simulink model "ee_asm_generator_fourier"  (R2021a)
settings: Solver=ode4  StartTime=0.0  StopTime=Wf.time(end)  FixedStep=1e-2  MaxStep=1e-4  RelTol=1e-3  EnableMultiTasking=on
PreLoadFcn:
  | SRated = 150e3; % V*A
  | VRated = 440; % V
  | FRated = 60; % Hz
  | 
  | QNominal = sin(acos(0.8))*SRated;
  | QPerPhase = QNominal / 3;
  | 
  | IPerPhase = QPerPhase/VRated;
  | Xc = VRated/IPerPhase;
  | reactiveCompensationCapacitance = 1/(2*pi*FRated*Xc);
  | 
  | clear( 'QNominal', 'QPerPhase', 'IPerPhase', 'Xc' );
StopFcn:
  | ee_addSimlogTimeStamp(bdroot)
undefined symbols (not defined in the file): g_r, H, i, J, Wf
libraries: ee_lib x8, nesl_utility x4, fl_lib x3
CloseFcn:
  | try,close(h1_ee_asm_generator),end
  | clear h1_ee_asm_generator
  | 
  | clear simlog_ee_asm_generator
  | clear logsout_ee_asm_generator
Description:
  | Three-Phase Asynchronous Wind Turbine Generator
settings Model: SimulationMode=accelerator  Creator=The MathWorks, Inc.  LastModifiedBy=Pedro
settings SolverCC: AlgebraicLoopSolver=TrustRegion
settings DataIOCC: LimitDataPoints=on  MaxDataPoints=610000  SaveFormat=Array  SaveOutput=off  SignalLogging=off  DSMLogging=off  SaveTime=off  ReturnWorkspaceOutputs=off  SignalLoggingName=logsout_ee_asm_generator
settings OptimizationCC: LifeSpan=inf
settings DebuggingCC: UnderspecifiedInitializationDetection=Classic  MergeDetectMultiDrivingBlocksExec=none  SFUnexpectedBacktrackingDiag=warning  SFNoUnconditionalDefaultTransitionDiag=warning  SFExecutionAtInitializationDiag=none  SFMachineParentedDataDiag=warning  ArithmeticOperatorsInVariantConditions=warning
settings HardwareCC: ProdBitPerPointer=32  ProdBitPerSizeT=32  ProdBitPerPtrDiffT=32  ProdLargestAtomicFloat=None  ProdIntDivRoundTo=Undefined  ProdEndianess=Unspecified  ProdWordSize=32  ProdHWDeviceType=32-bit Generic
settings ModelReferenceCC: PropagateSignalLabelsOutOfModel=off
settings SFSimCC: SimUseLocalCustomCode=off  CustomCodeUndefinedFunction=UseInterfaceOnly
settings RTWCC: RTWUseLocalCustomCode=off
settings CodeAppCC: StateflowObjectComments=on
settings GRTTargetCC: TargetLangStandard=C89/C90 (ANSI)
settings ConfigComp: CovMetricSettings=dw  CovSaveCumulativeToWorkspaceVar=on  CovSaveSingleToWorkspaceVar=on  CovExternalEMLEnable=off  CovSFcnEnable=off
settings SimscapeCC: SimscapeLogType=all  SimscapeLogSimulationStatistics=on  SimscapeLogName=simlog_ee_asm_generator  SimscapeLogDataHistory=610000

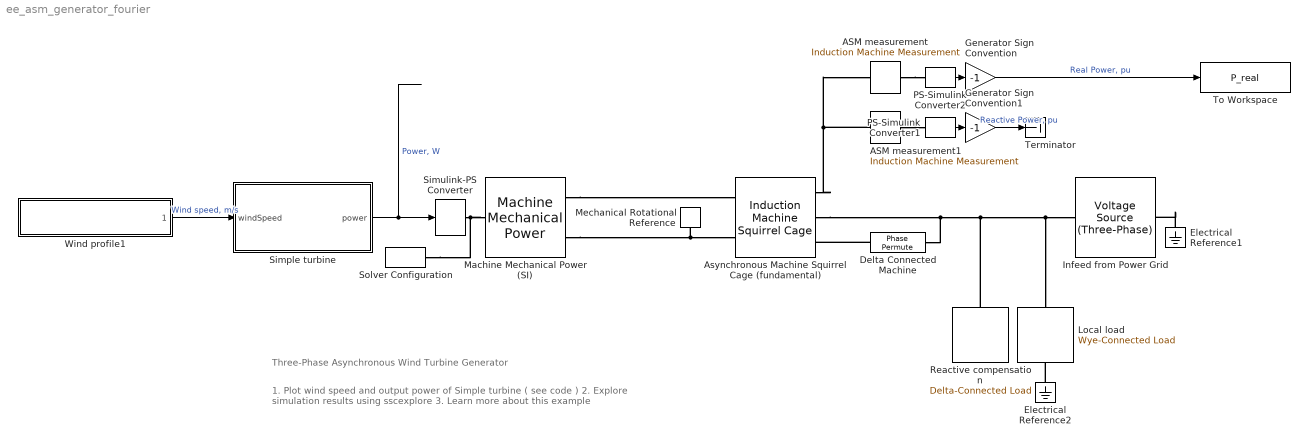
== system ee_asm_generator_fourier ==
  note: 1. Plot wind speed and output power of Simple turbine ( see code )
      | 2. Explore simulation results using sscexplore
      | 3. Learn more about this example
  note: Three-Phase Asynchronous Wind Turbine Generator
  ASM measurement : ee_lib/Electromechanical/Asynchronous/Induction Machine Measurement  output_idx=11
      settings: SourceProductBaseCode=PS  InternalSimscapePortConfiguration="{\"Bottom\":[],\"Left\":[{\"id\":\"pu_input\",\"label\":\"pu\",\"type\":\"input\"}],\"Right\":[{\"id\":\"pu_output\",\"label\":\"o\",\"type\":\"output\"}],\"Top\":[]}"
  ASM measurement1 : ee_lib/Electromechanical/Asynchronous/Induction Machine Measurement  output_idx=12
      settings: SourceProductBaseCode=PS  InternalSimscapePortConfiguration="{\"Bottom\":[],\"Left\":[{\"id\":\"pu_input\",\"label\":\"pu\",\"type\":\"input\"}],\"Right\":[{\"id\":\"pu_output\",\"label\":\"o\",\"type\":\"output\"}],\"Top\":[]}"
  Asynchronous Machine Squirrel Cage (fundamental) : ee_lib/Electromechanical/Asynchronous/Induction Machine Squirrel Cage  SRated=SRated V*A  VRated=VRated V  FRated=FRated Hz  nPolePairs=2  param_unit=ee.enum.unit.si  squirrel_cage=ee.enum.squirrelcage.Single  zero_sequence=ee.enum.park.zerosequence.include  Rs=0.25 Ohm  Xls=0.4 Ohm  pu_Rs=0.0258  pu_Lls=0.0413  Rrd=0.14 Ohm  Xlrd=0.41 Ohm  pu_Rrd=0.0145  pu_Llrd=0.0424  Rrd1=0.28 Ohm  Xlrd1=0.82 Ohm  Rrd2=0.28 Ohm  Xlrd2=0.82 Ohm  pu_Rrd1=0.0290  pu_Llrd1=0.0848  pu_Rrd2=0.0290  pu_Llrd2=0.0848  Xm=17 Ohm  pu_Lm=1.7562  X0=0.054 Ohm  pu_L0=0.0413  saturation_option=ee.enum.saturation.exclude  saturation_i=[0, 4, 9, 18, 25, 34, 50, 68, 95, 120] A  saturation_v=[0, 88, 154, 198, 220, 242, 264, 286, 308, 327] V  pu_saturation_i=[0, .176, .396, .792, 1.1, 1.496, 2.2, 2.992, 4.18, 5.28]  pu_saturation_v=[0, .4, .7, .9, 1, 1.1, 1.2, 1.3, 1.4, 1.4864]  initialization_option=ee.enum.asm.initialization.fluxvariables  connection_option=ee.enum.Connection.delta1  angular_position_specify=off  angular_position_priority=None  angular_position=0 deg  angular_position_nominal_specify=off  angular_position_nominal_unit=deg  angular_position_nominal_value=1  pu_psids_specify=off  pu_psids_priority=None  pu_psids=0  pu_psids_nominal_specify=off  pu_psids_nominal_unit=1  pu_psids_nominal_value=1  pu_psiqs_specify=off  pu_psiqs_priority=None  pu_psiqs=0  pu_psiqs_nominal_specify=off  pu_psiqs_nominal_unit=1  pu_psiqs_nominal_value=1  pu_psi0s_specify=off  pu_psi0s_priority=None  pu_psi0s=0  pu_psi0s_nominal_specify=off  pu_psi0s_nominal_unit=1  pu_psi0s_nominal_value=1  pu_psidr_specify=off  pu_psidr_priority=None  pu_psidr=0  pu_psidr_nominal_specify=off  pu_psidr_nominal_unit=1  pu_psidr_nominal_value=1  pu_psiqr_specify=off  pu_psiqr_priority=None  pu_psiqr=0  pu_psiqr_nominal_specify=off  pu_psiqr_nominal_unit=1  pu_psiqr_nominal_value=1  pu_psidr1_specify=off  pu_psidr1_priority=None  pu_psidr1=0  pu_psidr1_nominal_specify=off  pu_psidr1_nominal_unit=1  pu_psidr1_nominal_value=1  pu_psiqr1_specify=off  pu_psiqr1_priority=None  pu_psiqr1=0  pu_psiqr1_nominal_specify=off  pu_psiqr1_nominal_unit=1  pu_psiqr1_nominal_value=1  pu_psidr2_specify=off  pu_psidr2_priority=None  pu_psidr2=0  pu_psidr2_nominal_specify=off  pu_psidr2_nominal_unit=1  pu_psidr2_nominal_value=1  pu_psiqr2_specify=off  pu_psiqr2_priority=None  pu_psiqr2=0  pu_psiqr2_nominal_specify=off  pu_psiqr2_nominal_unit=1  pu_psiqr2_nominal_value=1  psids_specify=off  psids_priority=None  psids=0 Wb  psids_nominal_specify=off  psids_nominal_unit=Wb  psids_nominal_value=1  psiqs_specify=off  psiqs_priority=None  psiqs=0 Wb  psiqs_nominal_specify=off  psiqs_nominal_unit=Wb  psiqs_nominal_value=1  psi0s_specify=off  psi0s_priority=None  psi0s=0 Wb  psi0s_nominal_specify=off  psi0s_nominal_unit=Wb  psi0s_nominal_value=1  psidr_specify=off  psidr_priority=None  psidr=0 Wb  psidr_nominal_specify=off  psidr_nominal_unit=Wb  psidr_nominal_value=1  psiqr_specify=off  psiqr_priority=None  psiqr=0 Wb  psiqr_nominal_specify=off  psiqr_nominal_unit=Wb  psiqr_nominal_value=1  psidr1_specify=off  psidr1_priority=None  psidr1=0 Wb  psidr1_nominal_specify=off  psidr1_nominal_unit=Wb  psidr1_nominal_value=1  psiqr1_specify=off  psiqr1_priority=None  psiqr1=0 Wb  psiqr1_nominal_specify=off  psiqr1_nominal_unit=Wb  psiqr1_nominal_value=1  psidr2_specify=off  psidr2_priority=None  psidr2=0 Wb  psidr2_nominal_specify=off  psidr2_nominal_unit=Wb  psidr2_nominal_value=1  psiqr2_specify=off  psiqr2_priority=None  psiqr2=0 Wb  psiqr2_nominal_specify=off  psiqr2_nominal_unit=Wb  psiqr2_nominal_value=1  slip_specify=off  slip_priority=None  slip=0  slip_nominal_specify=off  slip_nominal_unit=1  slip_nominal_value=1  real_power_generated_specify=off  real_power_generated_priority=None  real_power_generated=0 W  real_power_generated_nominal_specify=off  real_power_generated_nominal_unit=W  real_power_generated_nominal_value=1  mechanical_power_consumed_specify=off  mechanical_power_consumed_priority=None  mechanical_power_consumed=0 W  mechanical_power_consumed_nominal_specify=off  mechanical_power_consumed_nominal_unit=W  mechanical_power_consumed_nominal_value=1
      settings: SourceProductBaseCode=PS  InternalSimscapePortConfiguration="{\"Bottom\":[],\"Left\":[{\"id\":\"R\",\"label\":\"R\",\"type\":\"foundation.mechanical.rotational.rotational\"},{\"id\":\"C\",\"label\":\"C\",\"type\":\"foundation.mechanical.rotational.rotational\"}],\"Right\":[{\"id\":\"pu_output\",\"label\":\"pu\",\"type\":\"output\"},{\"id\":\"N1\",\"label\":\"~1\",\"type\":\"foundation.electrical.three_phase\"},{\"id\":\"N2\",\"label\":\"~2\",\"type\":\"foundation.electrical.three_phase\"}],\"Top\":[]}"
  Delta Connected Machine : ee_lib/Connectors & References/Phase Permute
      settings: SourceProductBaseCode=PS  InternalSimscapePortConfiguration="{\"Bottom\":[],\"Left\":[{\"id\":\"N123\",\"label\":\"~123\",\"type\":\"foundation.electrical.three_phase\"}],\"Right\":[{\"id\":\"N231\",\"label\":\"~231\",\"type\":\"foundation.electrical.three_phase\"}],\"Top\":[]}"
  Electrical Reference1 : fl_lib/Electrical/Electrical Elements/Electrical Reference
  Electrical Reference2 : fl_lib/Electrical/Electrical Elements/Electrical Reference
  Generator Sign Convention : Gain  Gain=-1
  Generator Sign Convention1 : Gain  Gain=-1
  Infeed from Power Grid : ee_lib/Sources/Voltage Source (Three-Phase)  vline_rms=VRated V  shift=0 deg  freq=FRated Hz  impedance_option=3  SShortCircuit=1e6 V*A  XR=15  R=0.01 Ohm  L=3.97e-4 H  G_parasitic=0 1/Ohm  harmonic_option=0  harmonic_orders=[5, 7, 11, 13]  harmonic_ratios=[0.1, 0.1, 0.1, 0.1]  I_specify=off  I_priority=None  I=[ 0 0 0 ] A  I_nominal_specify=off  I_nominal_unit=A  I_nominal_value=1
      settings: SourceProductBaseCode=PS
  Local load : ee_lib/Passive/RLC Assemblies/Wye-Connected Load  parameterization=ee.enum.rlc.parameterization.ratedpower  component_structure=ee.enum.rlc.structure.R  component_structure_PQ=ee.enum.rlc.structure.R  R=1 Ohm  L=0.001 H  C=1e-6 F  R_parasitic=1e-6 Ohm  G_parasitic=1e-6 1/Ohm  VRated=VRated V  FRated=60 Hz  P=0.1 W  Qpos=100 V*A  Qneg=-100 V*A  Vmag0=2.4e+4 V  Vang0=0 deg  Freq0=60 Hz  R_parasitic_PQ=1e-6 Ohm  G_parasitic_PQ=1e-6 1/Ohm  IL_specify=on  IL_priority=High  IL=[ 0 0 0 ] A  IL_nominal_specify=off  IL_nominal_unit=A  IL_nominal_value=1  VC_specify=on  VC_priority=High  VC=[ 0 0 0 ] V  VC_nominal_specify=off  VC_nominal_unit=V  VC_nominal_value=1
      settings: SourceProductBaseCode=PS
  Machine Mechanical Power (SI) : ee_lib/Electromechanical/Mechanical/Machine Mechanical Power  power_sign=-1  SRated=SRated V*A  FRated=FRated Hz  nPolePairs=2  inputUnit=ee.enum.unit.si  torque_factor=2  inertia_option=1  J=H(i)%J(i)/(g_r(i)^2)%(25^2) kg*m^2  H=10 s*W/V/A  damper_option=2  D=39.0509 N*m/(rad/s)  pu_D=0.044  initialization_option=2  fMechanical0=30 Hz  fElectrical0=FRated Hz
      settings: SourceProductBaseCode=PS  InternalSimscapePortConfiguration="{\"Bottom\":[],\"Left\":[{\"id\":\"Pm\",\"label\":\"Pm\",\"type\":\"input\"}],\"Right\":[{\"id\":\"R\",\"label\":\"R\",\"type\":\"foundation.mechanical.rotational.rotational\"},{\"id\":\"C\",\"label\":\"C\",\"type\":\"foundation.mechanical.rotational.rotational\"}],\"Top\":[]}"
  Mechanical Rotational Reference : fl_lib/Mechanical/Rotational Elements/Mechanical Rotational Reference
  PS-Simulink Converter1 : nesl_utility/PS-Simulink Converter  PhysicalDomain=network_engine_domain  SubClassName=ps_output  LeftPortType=input  RightPortType=output  PseudoPeriodic=off  Frequencies=[]  Unit=1  AffineConversion=off
      settings: SourceProductBaseCode=PW,SS
  PS-Simulink Converter2 : nesl_utility/PS-Simulink Converter  PhysicalDomain=network_engine_domain  SubClassName=ps_output  LeftPortType=input  RightPortType=output  PseudoPeriodic=off  Frequencies=[]  Unit=1  AffineConversion=off
      settings: SourceProductBaseCode=PW,SS
  Reactive compensation : ee_lib/Passive/RLC Assemblies/Delta-Connected Load  parameterization=1  component_structure=3  component_structure_PQ=1  R=1 Ohm  L=0.001 H  C=reactiveCompensationCapacitance F  R_parasitic=1e-6 Ohm  G_parasitic=1e-6 1/Ohm  VRated=2.4e+4 V  FRated=60 Hz  P=1000 W  Qpos=100 V*A  Qneg=-100 V*A  Vmag0=2.4e+4 V  Vang0=0 deg  Freq0=60 Hz  R_parasitic_PQ=1e-6 Ohm  G_parasitic_PQ=1e-6 1/Ohm  IL_specify=on  IL_priority=High  IL=[ 0 0 0 ] A  IL_nominal_specify=off  IL_nominal_unit=A  IL_nominal_value=1  VC_specify=on  VC_priority=High  VC=[ 0 0 0 ] V  VC_nominal_specify=off  VC_nominal_unit=V  VC_nominal_value=1
      settings: SourceProductBaseCode=PS  InternalSimscapePortConfiguration="{\"Bottom\":[],\"Left\":[{\"id\":\"N\",\"label\":\"~\",\"type\":\"foundation.electrical.three_phase\"}],\"Right\":[],\"Top\":[]}"
  Simple turbine : MATLAB Function  TreatAsAtomicUnit=on  mask(Simple Turbine){ratedOutputPower=150000, cutInSpeed=3, ratedOutputSpeed=17, cutOutSpeed=23}
      mask prompts: ratedOutputPower "Rated output power, W"; cutInSpeed "Cut-in speed, m/s"; ratedOutputSpeed "Rated output speed, m/s"; cutOutSpeed "Cut-out speed, m/s"
      mask help:
      | This function implements a simple power versus wind speed characteristic to represent a wind turbine.
      |
      | Given an input of wind speed, m/s, the function outputs turbine power, W.
      |
      | The parameters must meet the following requirement:
      |
      | Cut-in speed < Rated output speed < Cut-out speed
  Simulink-PS Converter : nesl_utility/Simulink-PS Converter  PhysicalDomain=network_engine_domain  SubClassName=ps_input  LeftPortType=input  RightPortType=output  PseudoPeriodic=off  Frequencies=[]  NoiseDistribution=none  NoiseParameters=[]  Unit=1  AffineConversion=off  FilteringAndDerivatives=zero  SimscapeFilterOrder=1  InputFilterTimeConstant=0.001  UdotUserProvided=1
      settings: SourceProductBaseCode=PW,SS
  Solver Configuration : nesl_utility/Solver Configuration  PhysicalDomain=network_engine_domain  SubClassName=solver  LeftPortType=input  RightPortType=generic  Tones=[]  Harmonics=[]  SimulateNoise=off  Profile=off  UseLocalSampling=off  EnableSwitchedLinearOptims=on  FrequencyDomain=off  UseCCode=off  RelTol=0.001  AbsTol=1e-06  MinStep=1e-09  ToWorkspace=off  RevertToSquareIcSolve=off  NumHomotopyIterations=100  PhasorMode=off  PhasorModeNumHarmonics=1  DoDC=off  ResidualTolerance=1e-9  UseLocalSolver=on  LocalSolverChoice=NE_BACKWARD_EULER_ADVANCER  LocalSolverSampleTime=1e-2  DoFixedCost=on  MaxNonlinIter=3  MaxModeIter=2  ComputeImpulses=off  ImpulseIterations=2  LinearAlgebra=auto  EquationFormulation=NE_TIME_EF  DelaysMemoryBudget=1024  AutomaticFiltering=on  FilteringTimeConstant=0.001  PartitionStorageMethod=AS_NEEDED  PartitionMemoryBudget=1024  PartitionMethod=FAST
      settings: SourceProductBaseCode=PW,SS
  Terminator : Terminator
  To Workspace : ToWorkspace  VariableName=P_real  SaveFormat=Structure With Time  SampleTime=-1
  Wind profile1 : Subsystem
      mask init:
      | load power_V2G
      mask Display: plot(V2G.WINDTURBINE.time,V2G.WINDTURBINE.wind)
  wires:
  PS-Simulink Converter2/1 -> Generator Sign Convention/1
  Wind profile1/1(" ") -> Simple turbine/1(windSpeed)  "Wind speed, m/s"
  Simple turbine/1(power) -> Simulink-PS Converter/1  "Power, W"
  PS-Simulink Converter1/1 -> Generator Sign Convention1/1
  Generator Sign Convention/1 -> To Workspace/1  "Real Power, pu"
  Generator Sign Convention1/1 -> Terminator/1  "Reactive Power, pu"
  connections:
  Machine Mechanical Power (SI)/RConn2 -- Mechanical Rotational Reference/LConn1 -- Asynchronous Machine Squirrel Cage (fundamental)/LConn2
  Machine Mechanical Power (SI)/LConn1 -- Solver Configuration/RConn1 -- Simulink-PS Converter/RConn1
  Asynchronous Machine Squirrel Cage (fundamental)/RConn1 -- ASM measurement1/LConn1 -- ASM measurement/LConn1
  ASM measurement/RConn1 -- PS-Simulink Converter2/LConn1
  Delta Connected Machine/RConn1 -- Asynchronous Machine Squirrel Cage (fundamental)/RConn3
  Electrical Reference1/LConn1 -- Infeed from Power Grid/LConn1
  ASM measurement1/RConn1 -- PS-Simulink Converter1/LConn1
  Electrical Reference2/LConn1 -- Local load/RConn1
  Asynchronous Machine Squirrel Cage (fundamental)/RConn2 -- Delta Connected Machine/LConn1 -- Reactive compensation/LConn1 -- Infeed from Power Grid/RConn1 -- Local load/LConn1
  Machine Mechanical Power (SI)/RConn1 -- Asynchronous Machine Squirrel Cage (fundamental)/LConn1

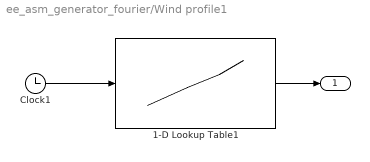
== system ee_asm_generator_fourier/Wind profile1 ==
  1-D Lookup Table1 : Lookup_n-D  NumberOfTableDimensions=1  BreakpointsForDimension1=Wf.time  BeginIndexSearchUsingPreviousIndexResult=on  Table=Wf.signals.values  ExtrapMethod=Clip  UseLastTableValue=on  InternalRulePriority=Speed  RndMeth=Simplest  InputSameDT=on
  Clock1 : Clock
  " " : Outport  VectorParamsAs1DForOutWhenUnconnected=off
  wires:
  Clock1/1 -> 1-D Lookup Table1/1
  1-D Lookup Table1/1 -> " "/1

== matlab function ee_asm_generator_fourier/Simple turbine ==
  data: windSpeed input; power output; ratedOutputPower parameter; cutInSpeed parameter; ratedOutputSpeed parameter; cutOutSpeed parameter
function power = simpleTurbine( windSpeed, ratedOutputPower, cutInSpeed, ratedOutputSpeed, cutOutSpeed ) %#codegen
%Simple Turbine
% This function implements a simple power versus wind speed characteristic
% to represent a wind turbine.
%
% Given an input of wind speed, m/s, the function outputs turbine power, W.
%
% The parameters must meet the following requirement:
%
% Cut-in speed < Rated output speed < Cut-out speed

% Check rated output power is greater than zero
if ~(ratedOutputPower > 0)
    error( 'Rated output power must be greater than zero.' );
end

% Check cut-in speed is less than rated output speed
if ~(cutInSpeed < ratedOutputSpeed)
    error( 'Cut-in speed must be less than rated output speed.' );
end

% Check rated output speed is less than cut-out speed
if ~(ratedOutputSpeed < cutOutSpeed)
    error( 'Rated output speed must be less than cut-out speed.' );
end

if windSpeed < cutInSpeed
    % Wind speed is less then cut-in speed, power output is zero
    power = 0;
elseif windSpeed < ratedOutputSpeed
    % Wind speed is greater than cut-in speed and less than rated output
    % speed, power output follows linear characteristic from zero to rated
    % power
    cutInGradient = ( ratedOutputPower / ( ratedOutputSpeed - cutInSpeed ) );
    power = cutInGradient * ( windSpeed - cutInSpeed );
elseif windSpeed < cutOutSpeed
    % Wind speed is greater than rated output speed and less than cut-out
    % speed, power output is limited to rated power
    power = ratedOutputPower;
else
    % Wind speed is greater than cut-out speed, power output is zero
    power = 0;
end
